simulink model "fly"  (R2016a)
settings: Solver=VariableStepAuto  StartTime=0.0  StopTime=100  RelTol=1e-3
undefined symbols (not defined in the file or in its folder): U_trim
libraries: X8_lib x1
settings Model: Creator=andreanv  LastModifiedBy=andreanv

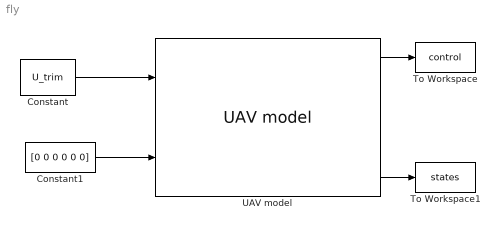
== system fly ==
  Constant : Constant  Value=U_trim
  Constant1 : Constant  Value=[0 0 0 0 0 0]
  To Workspace : ToWorkspace  VariableName=control  SaveFormat=Timeseries  SampleTime=-1
  To Workspace1 : ToWorkspace  VariableName=states  SaveFormat=Timeseries  SampleTime=-1
  UAV model : X8_lib/UAV model  param='x8_param'  pos0=[0,0,-100]  quat0=[1,0,0,0]  vel0=[0,0,0]  rate0=[0,0,0]  servoR_pos0=0  servoR_vel0=0  servoL_pos0=0  servoL_vel0=0  motor_speed0=0
  wires:
  Constant/1 -> UAV model/1
  Constant1/1 -> UAV model/2
  UAV model/1 -> To Workspace/1
  UAV model/4 -> To Workspace1/1
